simulink model "GalvoModel_thesis_v2_simpli"  (R2013a)
settings: Solver=ode45  StartTime=0.0  StopTime=10.0  RelTol=1e-3
undefined symbols (not defined in the file or in its folder): BEM, K1, K2, KTR, T1, T2
settings Model: Creator=mainster  LastModifiedBy=mainster
settings DebuggingCC: SolverPrmCheckMsg=none

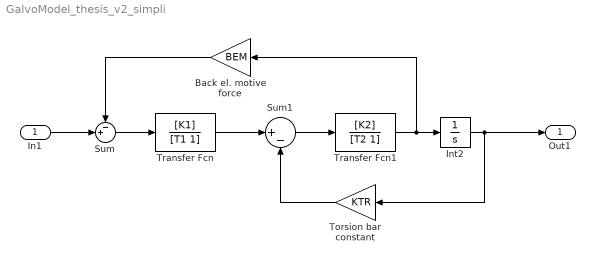
== system GalvoModel_thesis_v2_simpli ==
  In1 : Inport
  Back el. motive force : Gain  Gain=BEM
  Int2 : Integrator
  Sum : Sum  Inputs=-+|
  Sum1 : Sum  Inputs=|+-
  Torsion bar constant : Gain  Gain=KTR
  Transfer Fcn : TransferFcn  Numerator=[K1]  Denominator=[T1 1]
  Transfer Fcn1 : TransferFcn  Numerator=[K2]  Denominator=[T2 1]
  Out1 : Outport
  wires:
  In1/1 -> Sum/2
  Sum/1 -> Transfer Fcn/1
  Transfer Fcn/1 -> Sum1/1
  Sum1/1 -> Transfer Fcn1/1
  Transfer Fcn1/1 -> Back el. motive force/1, Int2/1
  Torsion bar constant/1 -> Sum1/2
  Int2/1 -> Out1/1, Torsion bar constant/1
  Back el. motive force/1 -> Sum/1
